simulink model "statecontrol2"  (R2022b)
settings: Solver=VariableStepAuto  StartTime=0.0  StopTime=0.5  FixedStep=1e-3  RelTol=1e-3
model workspace (MAT data in the model file):
  CC = [-1 -1]
values from neighbouring files (symbols this model uses):
  A = [-5 2 3 0 0 0 ... (first row only)    [retest004.m]    (also in retest007.m = [0	1	0	0)
  Brf = [-0.00130142918674408 ... (first row only)    [retest007.m]
  Bru = eye(6)    [retest004.m]    (also in retest007.m = [1.30358515621439e-08	1.30358515745248e-08)
  C = [1,0,0,0,0,0]    [retest004.m]    (also in retest007.m = [16.0376601050147	0.425434196872911	-35.4185444812321	-0.584)
  U0 = wa_0    [retest004.m]    (also in retest007.m)
undefined symbols (not defined in the file or in its folder): sigbuilder_block
libraries: simulink x3, dspsrcs4 x1
settings Model: Creator=Administrator  LastModifiedBy=NINGMEI

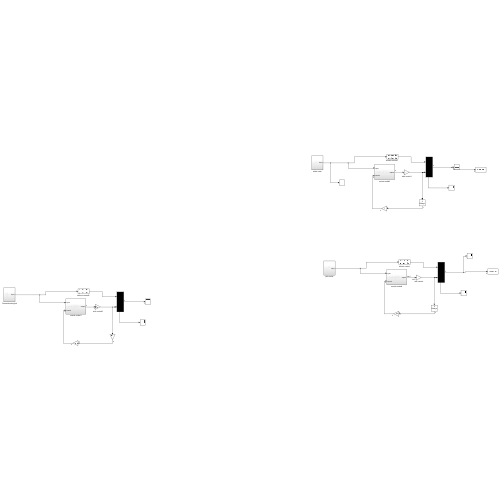
[thumbnail: Simulink's stored preview of the top-level diagram]
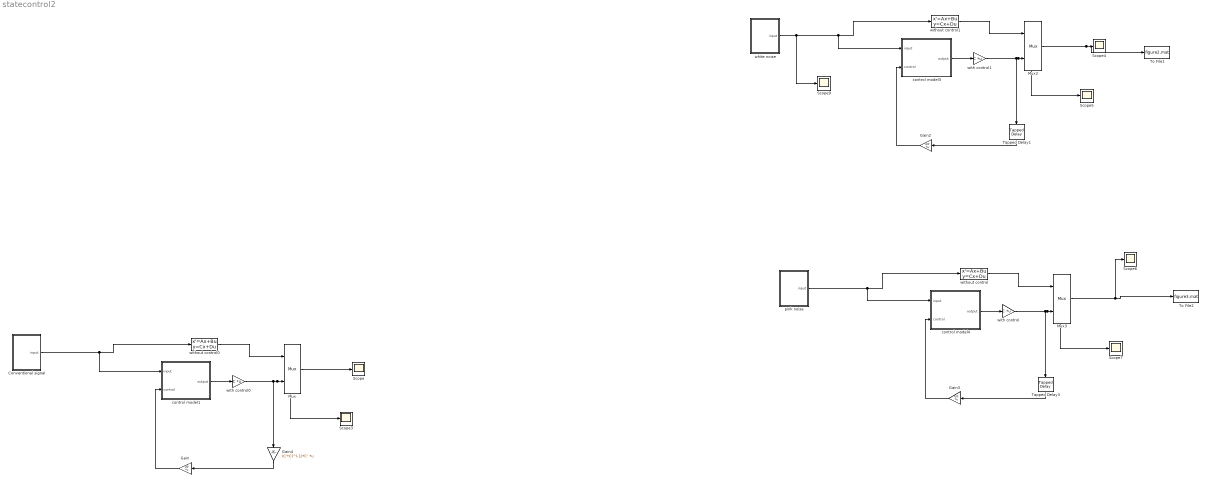
== system statecontrol2 ==
  " with control" : Gain  Gain=C  Multiplication=Matrix(K*u)
  " with control0" : Gain  Gain=C  Multiplication=Matrix(K*u)
  " with control1" : Gain  Gain=C  Multiplication=Matrix(K*u)
  Conventional signal : Subsystem
  Gain : Gain  Gain=U0'  Multiplication=Matrix(K*u)
  Gain2 : Gain  Gain=U0'  Multiplication=Matrix(K*u)
  Gain3 : Gain  Gain=U0'  Multiplication=Matrix(K*u)
  Gain4 : Gain  Gain=(C'*C)^(-1)*C'  Multiplication=Matrix(K*u)
  Mux : Mux  Inputs=2
  Mux2 : Mux  Inputs=2
  Mux3 : Mux  Inputs=2
  Scope{,3..7,9} (7 alike) : Scope
  Tapped Delay1 : simulink/Discrete/Tapped Delay  vinit=0.0  samptime=0.00025  NumDelays=4  DelayOrder=Oldest  includeCurrent=off
  Tapped Delay3 : simulink/Discrete/Tapped Delay  vinit=0.0  samptime=0.00025  NumDelays=4  DelayOrder=Oldest  includeCurrent=off
  To File1 : ToFile  Filename=figure2.mat  SaveFormat=Timeseries
  To File2 : ToFile  Filename=figure3.mat  SaveFormat=Timeseries
  control model1 : Subsystem
  control model3 : Subsystem
  control model4 : Subsystem
  pink noise : Subsystem
  white noise : Subsystem
  "without control " : StateSpace  A=A  B=Brf  C=C  D=0  InitialCondition=0
  "without control0 " : StateSpace  A=A  B=Brf  C=C  D=0  InitialCondition=0
  "without control1 " : StateSpace  A=A  B=Brf  C=C  D=0  InitialCondition=0
  wires:
  " with control0"/1 -> Scope3/1, Mux/2, Gain4/1
  control model1/1(output) -> " with control0"/1
  Mux/1 -> Scope/1
  Gain4/1 -> Gain/1
  "without control0 "/1 -> Mux/1
  Gain/1 -> control model1/2(control)
  Conventional signal/1(input) -> control model1/1(input), "without control0 "/1
  Gain2/1 -> control model3/2(control)
  "without control1 "/1 -> Mux2/1
  control model3/1(output) -> " with control1"/1
  white noise/1(input) -> control model3/1(input), "without control1 "/1, Scope9/1
  " with control1"/1 -> Scope5/1, Mux2/2, Tapped Delay1/1
  Mux2/1 -> To File1/1, Scope4/1
  Tapped Delay1/1 -> Gain2/1
  Gain3/1 -> control model4/2(control)
  "without control "/1 -> Mux3/1
  control model4/1(output) -> " with control"/1
  pink noise/1(input) -> control model4/1(input), "without control "/1
  " with control"/1 -> Scope7/1, Mux3/2, Tapped Delay3/1
  Mux3/1 -> To File2/1, Scope6/1
  Tapped Delay3/1 -> Gain3/1

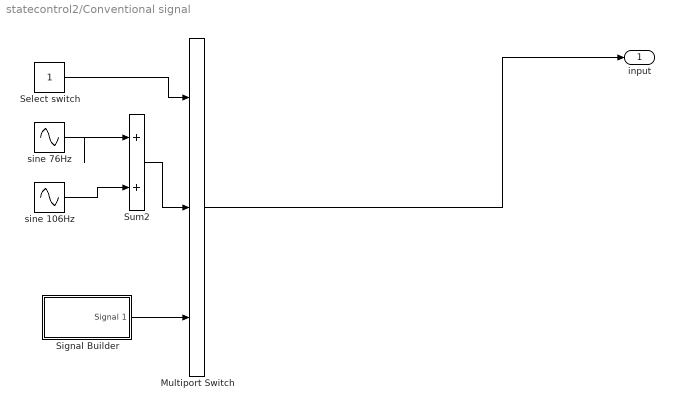
== system statecontrol2/Conventional signal ==
  Multiport Switch : MultiPortSwitch  Inputs=2  SaturateOnIntegerOverflow=off  InputSameDT=off
  Select switch : Constant
  Signal Builder : Subsystem  Tag=STV Subsys  LoadFcn=sigbuilder_block('load');  StartFcn=sigbuilder_block('start');  StopFcn=sigbuilder_block('stop');  ClipboardFcn=sigbuilder_block('clipboard');  mask(Sigbuilder block){tuvar=[0:10]}
      mask help: Simulink:masks:SigbuilderBlock_MD
      mask init:
      | if ~strcmp(get_param(bdroot(gcbh),'SimulationStatus'),'stopped') tuvar = sigbuilder_block('maskInit'); end
      settings: CopyFcn=sigbuilder_block('copy');  DeleteFcn=sigbuilder_block('delete');  ModelCloseFcn=sigbuilder_block('modelClose');  PreSaveFcn=sigbuilder_block('preSave');  PauseFcn=sigbuilder_block('pause');  ContinueFcn=sigbuilder_block('continue');  NameChangeFcn=sigbuilder_block('namechange');  OpenFcn=sigbuilder_block('open',[230.897 85.6552 549.931 396.621 ]);  CloseFcn=sigbuilder_block('close');
      mask Display: plot(0, 0, 100, 100,[2, 2, 32, 32, 2], [68, 8, 8, 68, 68],[32, 2], [38, 38], [32, 19, 2],[53, 60, 44], [32, 17, 17, 2],[16, 16, 31, 31]);txt = getActiveGroup(gcbh);text(2, 100, txt,'verticalAlignment', 'top');
  Sum2 : Sum  Inputs=|++
  sine 106Hz : Sin  Amplitude=0.5  Frequency=2*100*pi*1.06  SampleTime=0.001
  sine 76Hz : Sin  Amplitude=0.5  Frequency=2*100*pi*0.76  SampleTime=0.001
  input : Outport
  wires:
  Select switch/1 -> Multiport Switch/1
  sine 76Hz/1 -> Sum2/1
  Signal Builder/1(Signal 1) -> Multiport Switch/3
  sine 106Hz/1 -> Sum2/2
  Sum2/1 -> Multiport Switch/2
  Multiport Switch/1 -> input/1

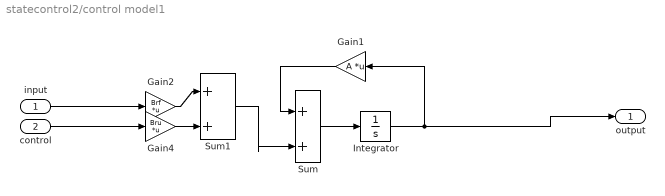
== system statecontrol2/control model1 ==
  input : Inport
  control : Inport  Port=2
  Gain1 : Gain  Gain=A  Multiplication=Matrix(K*u)
  Gain2 : Gain  Gain=Brf  Multiplication=Matrix(K*u)
  Gain4 : Gain  Gain=Bru  Multiplication=Matrix(K*u)
  Integrator : Integrator
  Sum : Sum  Inputs=|++
  Sum1 : Sum  Inputs=|++
  output : Outport
  wires:
  Gain1/1 -> Sum/1
  Sum/1 -> Integrator/1
  Integrator/1 -> output/1, Gain1/1
  input/1 -> Gain2/1
  control/1 -> Gain4/1
  Sum1/1 -> Sum/2
  Gain4/1 -> Sum1/2
  Gain2/1 -> Sum1/1

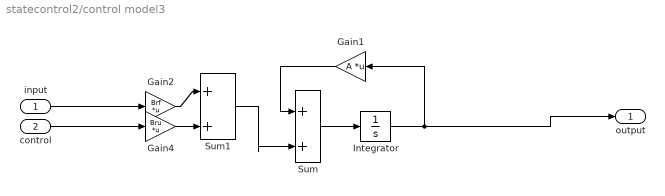
== system statecontrol2/control model3 ==
  input : Inport
  control : Inport  Port=2
  Gain1 : Gain  Gain=A  Multiplication=Matrix(K*u)
  Gain2 : Gain  Gain=Brf  Multiplication=Matrix(K*u)
  Gain4 : Gain  Gain=Bru  Multiplication=Matrix(K*u)
  Integrator : Integrator
  Sum : Sum  Inputs=|++
  Sum1 : Sum  Inputs=|++
  output : Outport
  wires:
  Gain1/1 -> Sum/1
  Sum/1 -> Integrator/1
  Integrator/1 -> output/1, Gain1/1
  input/1 -> Gain2/1
  control/1 -> Gain4/1
  Sum1/1 -> Sum/2
  Gain4/1 -> Sum1/2
  Gain2/1 -> Sum1/1

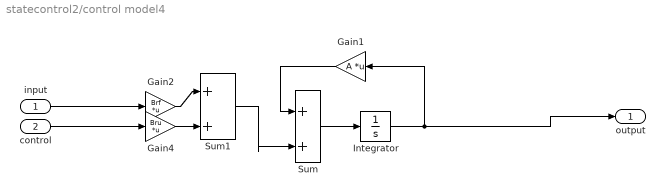
== system statecontrol2/control model4 ==
  input : Inport
  control : Inport  Port=2
  Gain1 : Gain  Gain=A  Multiplication=Matrix(K*u)
  Gain2 : Gain  Gain=Brf  Multiplication=Matrix(K*u)
  Gain4 : Gain  Gain=Bru  Multiplication=Matrix(K*u)
  Integrator : Integrator
  Sum : Sum  Inputs=|++
  Sum1 : Sum  Inputs=|++
  output : Outport
  wires:
  Gain1/1 -> Sum/1
  Sum/1 -> Integrator/1
  Integrator/1 -> output/1, Gain1/1
  input/1 -> Gain2/1
  control/1 -> Gain4/1
  Sum1/1 -> Sum/2
  Gain4/1 -> Sum1/2
  Gain2/1 -> Sum1/1

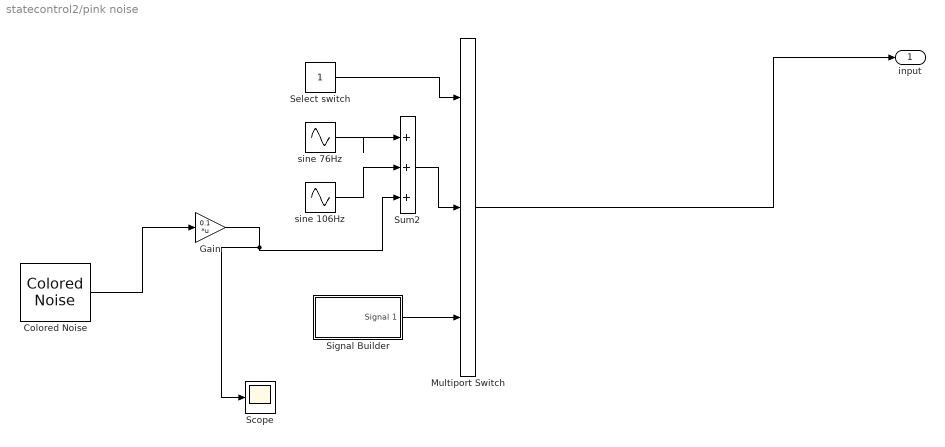
== system statecontrol2/pink noise ==
  Colored Noise : dspsrcs4/Colored Noise  Color=pink  InverseFrequencyPower=1  BoundedOutput=off  NumChannels=1  OutputDataType=double  SamplesPerFrame=1  SampleTime=0.001  RandomStream=mt19937ar with seed  Seed=67  SimulateUsing=Interpreted execution
      settings: LibrarySourceBlock=audiosources/Colored Noise
  Gain : Gain  Gain=0.1  Multiplication=Matrix(K*u)
  Multiport Switch : MultiPortSwitch  Inputs=2  SaturateOnIntegerOverflow=off  InputSameDT=off
  Scope : Scope
  Select switch : Constant
  Signal Builder : Subsystem  Tag=STV Subsys  LoadFcn=sigbuilder_block('load');  StartFcn=sigbuilder_block('start');  StopFcn=sigbuilder_block('stop');  ClipboardFcn=sigbuilder_block('clipboard');  mask(Sigbuilder block){tuvar=[0:10]}
      mask help: Simulink:masks:SigbuilderBlock_MD
      mask init:
      | if ~strcmp(get_param(bdroot(gcbh),'SimulationStatus'),'stopped') tuvar = sigbuilder_block('maskInit'); end
      settings: CopyFcn=sigbuilder_block('copy');  DeleteFcn=sigbuilder_block('delete');  ModelCloseFcn=sigbuilder_block('modelClose');  PreSaveFcn=sigbuilder_block('preSave');  PauseFcn=sigbuilder_block('pause');  ContinueFcn=sigbuilder_block('continue');  NameChangeFcn=sigbuilder_block('namechange');  OpenFcn=sigbuilder_block('open',[230.897 85.6552 549.931 396.621 ]);  CloseFcn=sigbuilder_block('close');
      mask Display: plot(0, 0, 100, 100,[2, 2, 32, 32, 2], [68, 8, 8, 68, 68],[32, 2], [38, 38], [32, 19, 2],[53, 60, 44], [32, 17, 17, 2],[16, 16, 31, 31]);txt = getActiveGroup(gcbh);text(2, 100, txt,'verticalAlignment', 'top');
  Sum2 : Sum  Inputs=|+++
  sine 106Hz : Sin  Amplitude=0.5  Frequency=2*100*pi*1.06  SampleTime=0.001
  sine 76Hz : Sin  Amplitude=0.5  Frequency=2*100*pi*0.76  SampleTime=0.001
  input : Outport
  wires:
  Select switch/1 -> Multiport Switch/1
  sine 76Hz/1 -> Sum2/1
  Signal Builder/1(Signal 1) -> Multiport Switch/3
  sine 106Hz/1 -> Sum2/2
  Sum2/1 -> Multiport Switch/2
  Multiport Switch/1 -> input/1
  Colored Noise/1 -> Gain/1
  Gain/1 -> Scope/1, Sum2/3

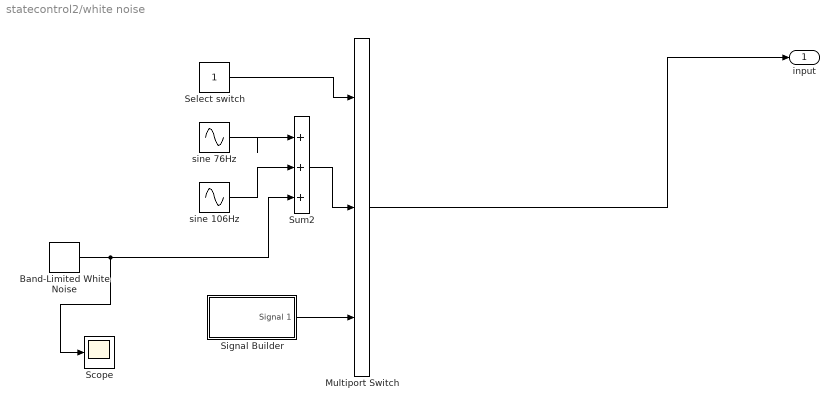
== system statecontrol2/white noise ==
  Band-Limited White Noise : simulink/Sources/Band-Limited White Noise  Cov=[0.00001]  Ts=0.001  seed=[23341]
  Multiport Switch : MultiPortSwitch  Inputs=2  SaturateOnIntegerOverflow=off  InputSameDT=off
  Scope : Scope
  Select switch : Constant
  Signal Builder : Subsystem  Tag=STV Subsys  LoadFcn=sigbuilder_block('load');  StartFcn=sigbuilder_block('start');  StopFcn=sigbuilder_block('stop');  ClipboardFcn=sigbuilder_block('clipboard');  mask(Sigbuilder block){tuvar=[0:10]}
      mask help: Simulink:masks:SigbuilderBlock_MD
      mask init:
      | if ~strcmp(get_param(bdroot(gcbh),'SimulationStatus'),'stopped') tuvar = sigbuilder_block('maskInit'); end
      settings: CopyFcn=sigbuilder_block('copy');  DeleteFcn=sigbuilder_block('delete');  ModelCloseFcn=sigbuilder_block('modelClose');  PreSaveFcn=sigbuilder_block('preSave');  PauseFcn=sigbuilder_block('pause');  ContinueFcn=sigbuilder_block('continue');  NameChangeFcn=sigbuilder_block('namechange');  OpenFcn=sigbuilder_block('open',[230.897 85.6552 549.931 396.621 ]);  CloseFcn=sigbuilder_block('close');
      mask Display: plot(0, 0, 100, 100,[2, 2, 32, 32, 2], [68, 8, 8, 68, 68],[32, 2], [38, 38], [32, 19, 2],[53, 60, 44], [32, 17, 17, 2],[16, 16, 31, 31]);txt = getActiveGroup(gcbh);text(2, 100, txt,'verticalAlignment', 'top');
  Sum2 : Sum  Inputs=|+++
  sine 106Hz : Sin  Amplitude=0.5  Frequency=2*100*pi*1.06  SampleTime=0.001
  sine 76Hz : Sin  Amplitude=0.5  Frequency=2*100*pi*0.76  SampleTime=0.001
  input : Outport
  wires:
  Select switch/1 -> Multiport Switch/1
  sine 76Hz/1 -> Sum2/1
  Signal Builder/1(Signal 1) -> Multiport Switch/3
  sine 106Hz/1 -> Sum2/2
  Sum2/1 -> Multiport Switch/2
  Multiport Switch/1 -> input/1
  Band-Limited White Noise/1 -> Scope/1, Sum2/3

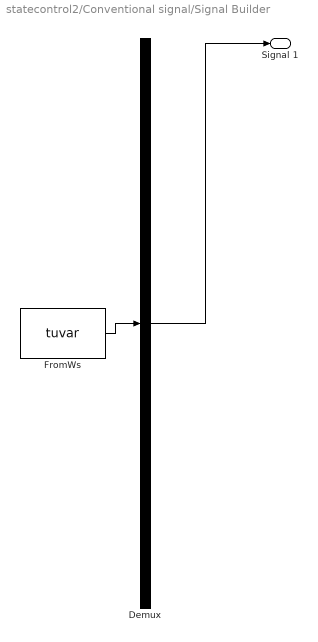
== system statecontrol2/Conventional signal/Signal Builder ==
  Demux : Demux  Tag=STV Demux  Outputs=1
      settings: DisplayOption=none
  FromWs : FromWorkspace  Tag=STV FromWs  VariableName=tuvar
      SigBuilderData=|
      | common.afterFinalStr = 'Extrapolate'
      | common.sampleTime = 0
      | dataSet.timeRange = [0 10]
      | dataSet.name = 'Group 1'
      | sbobj.Groups.Name = 'Group 1'
      | sbobj.Groups.Signals.Name = 'Signal 1'
      | sbobj.Groups.Signals.XData = [0 0.1 0.1 0.1001 0.1001 10]
      | sbobj.Groups.Signals.YData = [0 0 1 1 0 0]
  Signal 1 : Outport  Tag=STV Outport
  wires:
  Demux/1 -> Signal 1/1
  FromWs/1 -> Demux/1

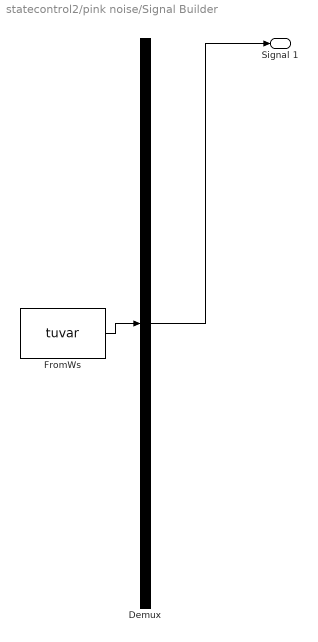
== system statecontrol2/pink noise/Signal Builder ==
  Demux : Demux  Tag=STV Demux  Outputs=1
      settings: DisplayOption=none
  FromWs : FromWorkspace  Tag=STV FromWs  VariableName=tuvar
      SigBuilderData=|
      | common.afterFinalStr = 'Extrapolate'
      | common.sampleTime = 0
      | dataSet.timeRange = [0 10]
      | dataSet.name = 'Group 1'
      | sbobj.Groups.Name = 'Group 1'
      | sbobj.Groups.Signals.Name = 'Signal 1'
      | sbobj.Groups.Signals.XData = [0 0.1 0.1 0.1001 0.1001 10]
      | sbobj.Groups.Signals.YData = [0 0 1 1 0 0]
  Signal 1 : Outport  Tag=STV Outport
  wires:
  Demux/1 -> Signal 1/1
  FromWs/1 -> Demux/1

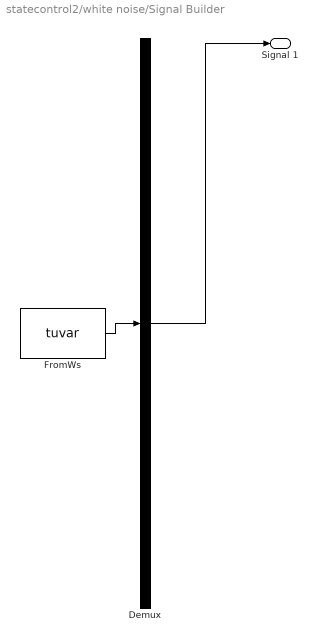
== system statecontrol2/white noise/Signal Builder ==
  Demux : Demux  Tag=STV Demux  Outputs=1
      settings: DisplayOption=none
  FromWs : FromWorkspace  Tag=STV FromWs  VariableName=tuvar
      SigBuilderData=|
      | common.afterFinalStr = 'Extrapolate'
      | common.sampleTime = 0
      | dataSet.timeRange = [0 10]
      | dataSet.name = 'Group 1'
      | sbobj.Groups.Name = 'Group 1'
      | sbobj.Groups.Signals.Name = 'Signal 1'
      | sbobj.Groups.Signals.XData = [0 0.1 0.1 0.1001 0.1001 10]
      | sbobj.Groups.Signals.YData = [0 0 1 1 0 0]
  Signal 1 : Outport  Tag=STV Outport
  wires:
  Demux/1 -> Signal 1/1
  FromWs/1 -> Demux/1
